simulink model "Elevator_RQ"  (R2020a)
settings: Solver=FixedStepAuto  StartTime=0.0  StopTime=inf  RelTol=1e-3
undefined symbols (not defined in the file): DiscIntNeverNeededParam
settings Model: EnablePacing=on  Creator=jatin  LastModifiedBy=jatin
settings ConfigComp: DVMode=PropertyProving  DVMaxProcessTime=NaN  DVTestSuiteOptimization=Auto  DVDetectOutOfBounds=on

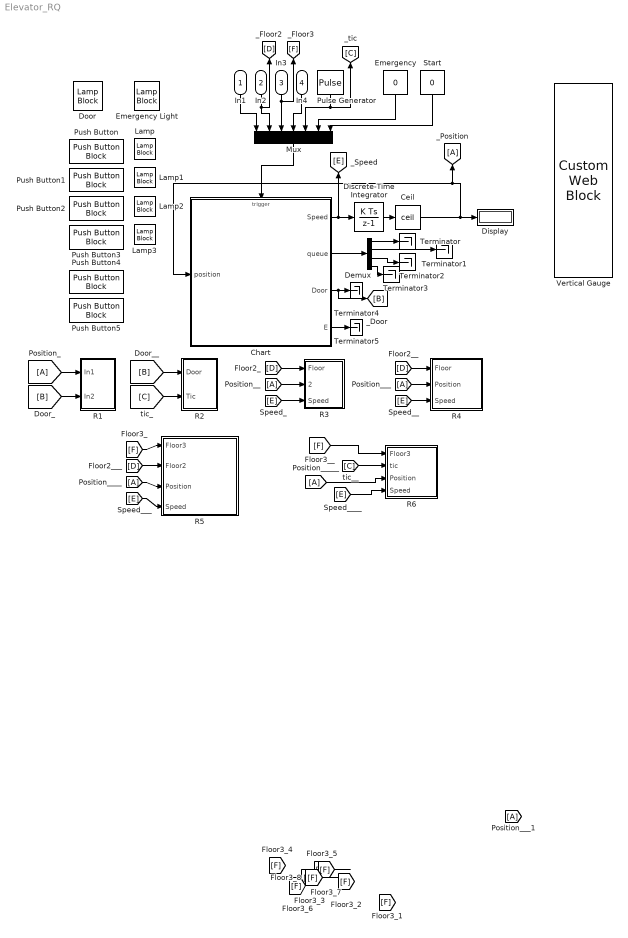
== system Elevator_RQ ==
  In1 : Inport
  In2 : Inport  Port=2
  In3 : Inport  Port=3
  In4 : Inport  Port=4
  Ceil : Rounding  Operator=ceil
  Chart : Stateflow chart  TreatAsAtomicUnit=on
  Demux : Demux
  Discrete-Time Integrator : DiscreteIntegrator  InitialCondition=0.001  SampleTime=-1  ICPrevOutput=DiscIntNeverNeededParam  ICPrevScaledInput=DiscIntNeverNeededParam
  Display : Display
  Door : LampBlock
  Emergency : Constant  Value=0
  Emergency Light : LampBlock
  Lamp{,1..3} (4 alike) : LampBlock
  Mux : Mux  Inputs=7
  Pulse Generator : DiscretePulseGenerator  PulseType=Time based  Period=1  PulseWidth=50
  Push Button : PushButtonBlock  ButtonText=floor1
  Push Button1 : PushButtonBlock  ButtonText=floor2
  Push Button2 : PushButtonBlock  ButtonText=floor3
  Push Button3 : PushButtonBlock  ButtonText=floor4
  Push Button4 : PushButtonBlock  ButtonText=Emergency
  Push Button5 : PushButtonBlock  ButtonText=Start
  R1 : Subsystem
  R2 : Subsystem
  R3 : Subsystem
  R4 : Subsystem
  R5 : Subsystem
  R6 : Subsystem
  Start : Constant  Value=0
  Terminator{,1..5} (6 alike) : Terminator
  Vertical Gauge : CustomWebBlock  ShowInitialText=on  Configuration="{\"components\":[{\"name\":\"LinearScaleComponent\",\"settings\":{\"bounds\":{\"max\":4,\"min\":1,\"tickInterval\":\"auto\"},\"labelColor\":[250,245,199],\"labelFont\":{\"font\":\"Arial\",\"fontSize\":12},\"labelTransparency\":1,\"needleImage\":{\"size\":[21,75],\"src\":\"data:image\\/svg+xml;base64,PHN2ZyB4bWxucz0iaHR0cDovL3d3dy53My5vcmcvMjAwMC9zdmciIHhtbG5zOnhsaW5rPSJodHRwOi8vd3d3LnczLm9yZy8xOTk5L3hsaW5rIiB2aWV3Qm94PSIwIDAgMjEgNzUiPjxkZWZzPjxzdHlsZT4uY2xzLTF7ZmlsbDpub25lO30uY2xzLTJ7aXNvbGF0aW9uOmlzb2xhdGU7fS5jbHMtM3tjbGlwLXBhdGg6dXJsKCNjbGlwLXBhdGgpO30uY2xzLTR7b3BhY2l0eTowLjM7bWl4LWJsZW5kLW1vZGU6bXVsdGlwbHk7fS5jbHMtNXtmaWxsOiNlYjI2Mjk7fTwvc3R5bGU+PGNsaXBQYXRoIGlkPSJjbGlwLXBhdGgiIHRyYW5zZm9y ...(+1928 chars)\",\"srcOrientation\":\"horizontal\"},\"needleOffset\":[-0.01094391244870041,0],\"needleSize\":{\"height\":0.11960078534031414,\"width\":0.7589285714285714},\"position\":[0.015887605042016806,0.06986607142857143,0.8,0.9641544117647058],\"scaleColorSize\":0.24,\"scaleColors\":[],\"scaleColorsSize\":0.2,\"tickColor\":[250,245,200],\"tickTransparency\":1,\"valueBarColor\":[23,89,176],\"valueBarSize\":0.23,\"valueBarTransparency\":1}},{\"name\":\"BackgroundImageComponent\",\"settings\":{\"image\":{\"size\":[380,101],\"src\":\"data:image\\/svg+xml;base64,PHN2ZyB4bWxucz0iaHR0cDovL3d3dy53My5vcmcvMjAwMC9zdmciIHhtbG5zOnhsaW5rPSJodHRwOi8vd3d3LnczLm9yZy8xOTk5L3hsaW5rIiB2aWV3Qm94PSIwIDAgMzgwIDEwMSI+PGRlZnM+PHN0eWxlPi5jbHMtMXtmaWxsOnVybCgjbGluZWFyLWdyYWRpZW50KTt9LmNscy0ye2ZpbGw6dXJsKCNsaW5lYXItZ3JhZGllbnQtMik7fS5jbHMtM3tmaWxsOnVybCgjbGluZWFyLWdyYWRpZW50LTMpO308L3N0eWxlPjxsaW5lYXJHcmFkaWVudCBpZD0ibGluZWFyLWdyYWRpZW50IiB5MT0iNTAuNSIgeDI9IjM5OS4yOCIgeTI9IjUw ...(+2216 chars)\",\"srcOrientation\":\"horizontal\"},\"position\":[0,0,1,1],\"scaleMode\":\"0\"}}],\"settings\":{\"BindingType\":\"signal\",\"fixedAspectRatio\":\"on\",\"orientation\":\"vertical\"},\"type\":\"LinearGauge\"}"
  wires:
  Pulse Generator/1 -> Mux/5, [C]
  Mux/1 -> Chart/Trigger
  Chart/1(Speed) -> Discrete-Time Integrator/1, [E]
  Ceil/1 -> Chart/1(position), [A], Display/1
  Demux/1 -> Terminator/1
  Demux/2 -> Terminator1/1
  Demux/3 -> Terminator2/1
  Demux/4 -> Terminator3/1
  Chart/2(queue) -> Demux/1
  Emergency/1 -> Mux/6
  Start/1 -> Mux/7
  Chart/4(E) -> Terminator5/1
  In1/1 -> Mux/1
  In2/1 -> Mux/2, [D]
  In3/1 -> Mux/3, [F]
  In4/1 -> Mux/4
  Chart/3(Door) -> [B], Terminator4/1
  [A] -> R1/1(In1)
  [B] -> R1/2(In2)
  Discrete-Time Integrator/1 -> Ceil/1
  [B] -> R2/1(Door)
  [C] -> R2/2(Tic)
  [D] -> R3/1(Floor)
  [A] -> R3/2(Position)
  [E] -> R3/3(Speed)
  [D] -> R4/1(Floor)
  [A] -> R4/2(Position)
  [E] -> R4/3(Speed)
  [F] -> R5/1("\tFloor3")
  [D] -> R5/2(Floor2)
  [A] -> R5/3(Position)
  [E] -> R5/4(Speed)
  [F] -> ?
  [F] -> ?
  [F] -> R6/1(Floor3)
  [C] -> R6/2(tic)
  [A] -> R6/3(Position)
  [E] -> R6/4(Speed)

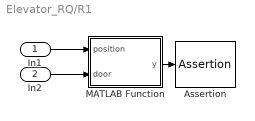
== system Elevator_RQ/R1 ==
  In1 : Inport
  In2 : Inport  Port=2
  Assertion : Assertion
  MATLAB Function : MATLAB Function  TreatAsAtomicUnit=on
  wires:
  In2/1 -> MATLAB Function/2(door)
  MATLAB Function/1(y) -> Assertion/1
  In1/1 -> MATLAB Function/1(position)

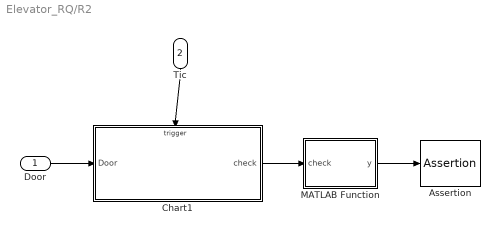
== system Elevator_RQ/R2 ==
  Door : Inport
  Tic : Inport  Port=2
  Assertion : Assertion
  Chart1 : Stateflow chart  TreatAsAtomicUnit=on
  MATLAB Function : MATLAB Function  TreatAsAtomicUnit=on
  wires:
  Tic/1 -> Chart1/Trigger
  Door/1 -> Chart1/1(Door)
  Chart1/1(check) -> MATLAB Function/1(check)
  MATLAB Function/1(y) -> Assertion/1

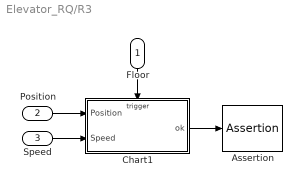
== system Elevator_RQ/R3 ==
  Floor : Inport
  Position : Inport  Port=2
  Speed : Inport  Port=3
  Assertion : Assertion
  Chart1 : Stateflow chart  TreatAsAtomicUnit=on
  wires:
  Position/1 -> Chart1/1(Position)
  Floor/1 -> Chart1/Trigger
  Speed/1 -> Chart1/2(Speed)
  Chart1/1(ok) -> Assertion/1

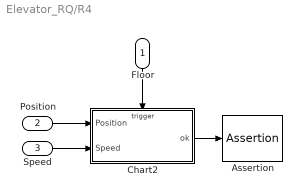
== system Elevator_RQ/R4 ==
  Floor : Inport
  Position : Inport  Port=2
  Speed : Inport  Port=3
  Assertion : Assertion
  Chart2 : Stateflow chart  TreatAsAtomicUnit=on
  wires:
  Floor/1 -> Chart2/Trigger
  Position/1 -> Chart2/1(Position)
  Speed/1 -> Chart2/2(Speed)
  Chart2/1(ok) -> Assertion/1

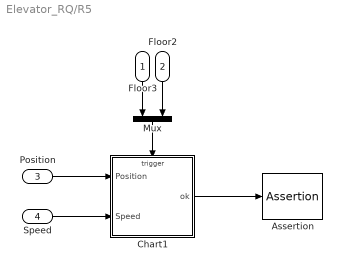
== system Elevator_RQ/R5 ==
  "\tFloor3" : Inport
  Floor2 : Inport  Port=2
  Position : Inport  Port=3
  Speed : Inport  Port=4
  Assertion : Assertion
  Chart1 : Stateflow chart  TreatAsAtomicUnit=on
  Mux : Mux  Inputs=2
  wires:
  "\tFloor3"/1 -> Mux/1
  Floor2/1 -> Mux/2
  Mux/1 -> Chart1/Trigger
  Speed/1 -> Chart1/2(Speed)
  Position/1 -> Chart1/1(Position)
  Chart1/1(ok) -> Assertion/1

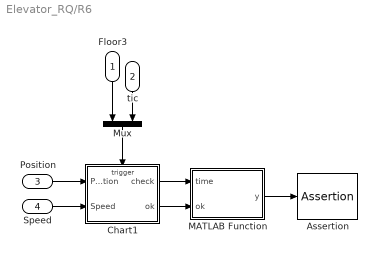
== system Elevator_RQ/R6 ==
  Floor3 : Inport
  tic : Inport  Port=2
  Position : Inport  Port=3
  Speed : Inport  Port=4
  Assertion : Assertion
  Chart1 : Stateflow chart  TreatAsAtomicUnit=on
  MATLAB Function : MATLAB Function  TreatAsAtomicUnit=on
  Mux : Mux  Inputs=2
  wires:
  tic/1 -> Mux/2
  Floor3/1 -> Mux/1
  Mux/1 -> Chart1/Trigger
  Position/1 -> Chart1/1(Position)
  Speed/1 -> Chart1/2(Speed)
  Chart1/1(check) -> MATLAB Function/1(time)
  Chart1/2(ok) -> MATLAB Function/2(ok)
  MATLAB Function/1(y) -> Assertion/1

== stateflow chart Elevator_RQ/R2/Chart1 ==
  state Door_open
  state counter
    on tic: check=check+1;
  state Door_close
  (default) -> Door_open : {check=0;}
  Door_open -> counter : [Door==1]
  counter -> Door_close : [Door==0]
  data: Door input; check output
  events: tic input RISING_EDGE_EVENT

== matlab function Elevator_RQ/R1/MATLAB Function ==
  data: position input; y output; door input
function y = fcn(position,door)
if (position~=1 || position~=2 || position~=3 || position~=4) && door==1
    y=0;
else
    y=1;
end

== stateflow chart Elevator_RQ/Chart ==
  settings: executeAtInitialization=1
  state Init
    on floor1: queue(1)=1;new_dest=1;
    on floor2: queue(2)=1;new_dest=2;
    on floor3: queue(3)=1;new_dest=3;
    on floor4: queue(4)=1;new_dest=4;
    state Up
      Speed=0.2;
    state Door
      Speed=0;Door=1;
      (default) -> (junction 51)
      (junction 51) -> (junction 52) [order 1] : [flag==1]{queue(dest)=0;}
      (junction 51) -> (junction 53) [order 2] : [flag==0]{queue(new_dest)=0;new_dest=0;}
    state Idle_state
    state Emergency
      Speed=0;
    state Down
      Speed=-0.2;
    Idle_state -> Door [order 4] : [queue(position)]
    Up -> Door [order 2] : [(new_dest<dest && new_dest>=position) && position>=new_dest-0.02]{flag=0;}
    Idle_state -> Up [order 2] : [floor_check==1]
    Up -> Door [order 3] : [position>=dest-0.02]{flag=1;}
    Up -> Emergency [order 1] : Emergency{u=1;E=1;}
    Emergency -> Up [order 2] : Start[u==1]{u=0;E=0;}
    (default) -> Idle_state
    Door -> Emergency [order 1] : Emergency{do=1;E=1;}
    Idle_state -> Emergency [order 1] : Emergency{i=1;E=1;}
    Emergency -> Idle_state [order 1] : Start[i==1]{E=0;i=0;}
    Emergency -> Door [order 3] : Start[do==1]{do=0;E=0;}
    Door -> Idle_state [order 2] : [after(5,sec)]{Door=0;}
    Down -> Emergency [order 3] : Emergency{d=1;E=1;}
    Emergency -> Down [order 4] : Start[d==1]{d=0;E=0;}
    Idle_state -> Down [order 3] : [floor_check==0]
    Down -> Door [order 1] : [position<=dest+0.02]{flag=1;}
    Down -> Door [order 2] : [(new_dest>dest && new_dest<=position) && position<=new_dest+0.02]{flag=0;}
  (default) -> Init : {Speed=0;queue(1)=0;E=0;new_dest=0;i=0;u=0;d=0;do=0;}
  data: out function_output; Speed output; dest local; position input; new_dest local; queue output double size=[1 4]; flag local; Door output; E output; d local; do local; i local; u local
  events: floor1 input RISING_EDGE_EVENT; floor2 input RISING_EDGE_EVENT; floor3 input RISING_EDGE_EVENT; floor4 input RISING_EDGE_EVENT; tic input RISING_EDGE_EVENT; Emergency input RISING_EDGE_EVENT; Start input RISING_EDGE_EVENT
  function out = floor_check:
    | function out = floor_check
    | if queue(2)&& position<2
    |     dest=2;
    |     out=1;  
    | elseif queue(3) && position<3
    |     dest=3;
    |     out=1;
    | elseif queue(4)&& position~=4
    |     dest=4;
    |     out=1;
    | elseif queue(1)&& position~=1
    |     dest=1;
    |     out=0;
    | elseif queue(2)&& position>2
    |     dest=2;
    |     out=0;
    | elseif queue(3)&& position>3
    |     dest=3;
    |     out=0;
    | else
    |     out=-1;
    | end

== matlab function Elevator_RQ/R2/MATLAB Function ==
  data: check input; y output
function y = fcn(check)
if check<5
    y=0;
else
    y=1;
end

== stateflow chart Elevator_RQ/R3/Chart1 ==
  state OnFloorPress
  state StopAtFloor_2
    ok=1;
  state StopAtFloor
  state StopAtFloor2
    ok=0;
  (default) -> OnFloorPress : {ok=1;}
  StopAtFloor -> StopAtFloor_2 : [Speed==0 && Position==2]
  OnFloorPress -> StopAtFloor [order 1] : Floor
  OnFloorPress -> StopAtFloor2 [order 2] : [Speed==0 && Position==2]
  data: Position input; ok output; Speed input
  events: Floor input RISING_EDGE_EVENT

== stateflow chart Elevator_RQ/R5/Chart1 ==
  state Check
  state Reached_A
    ok=0;
  state FloorA
  state FloorB
  state Floor_A
  state Reached_B
    ok=1;
  state Reached__A
  (default) -> Check : {ok=1;}
  Check -> FloorB : Floor3
  FloorB -> FloorA [order 1] : Floor2[Position>2]
  FloorA -> Reached_A : [Position==2 && Speed==0]
  FloorB -> Floor_A [order 2] : Floor2[Position<=2]
  FloorB -> Reached_B [order 3] : [Position==3 && Speed==0]
  Floor_A -> Reached__A : [Position==2 && Speed==0]
  Reached__A -> Reached_B : [Position==3 &&Speed==0]
  data: Position input; Speed input; ok output
  events: Floor3 input RISING_EDGE_EVENT; Floor2 input RISING_EDGE_EVENT

== stateflow chart Elevator_RQ/R4/Chart2 ==
  state OnFloorPress
  state StopAtFloor_2
    ok=1;
  state StopAtFloor
  state CheckAgain
  state StopAtFloor2
    ok=0;
  state BackToFloor
  (default) -> OnFloorPress : {ok=1;}
  StopAtFloor_2 -> CheckAgain : [Position~=2 && Speed~=0]
  OnFloorPress -> StopAtFloor [order 1] : Floor
  StopAtFloor -> StopAtFloor_2 : [Speed==0 && Position==2]
  OnFloorPress -> StopAtFloor2 [order 2] : [Speed==0 && Position==2]
  CheckAgain -> BackToFloor : Floor
  BackToFloor -> StopAtFloor2 : [Speed==0 && Position==2]
  data: Position input; ok output; Speed input
  events: Floor input RISING_EDGE_EVENT

== stateflow chart Elevator_RQ/R6/Chart1 ==
  state Counter
    on tic: check=check+1;
  state Init
  state Reached
    ok=1;
  (default) -> Init : {ok=0;check=0;}
  Counter -> Reached : [Position==3 && Speed==0]
  Init -> Counter : Floor3
  data: Position input; Speed input; check output; ok output
  events: Floor3 input RISING_EDGE_EVENT; tic input RISING_EDGE_EVENT

== matlab function Elevator_RQ/R6/MATLAB Function ==
  data: time input; y output; ok input
function y = fcn(time,ok)
if time<26 && ok==1
    y=0;
else 
    y=1;
end
